simulink model "PTControl"  (Simulink 7.9)
settings: Solver=ode45  StartTime=0.0  StopTime=inf  RelTol=1e-3
PreLoadFcn:
  | FSE_Parameters
undefined symbols (not defined in the file or in its folder): TC_Decr_Gas, TC_Derivative, TC_Incr_Gas, TC_On, TC_Relay_Off, TC_Relay_On, TV_On, TV_Override
libraries: CarMaker4SL x33, simulink x5, simulink_extras x4
(part 2 of 3)

== system PTControl/CarMaker/IPG Vehicle/CarAndTrailer/Trailer/CreateBus Vhcl.Wheel.FL ==
  In1 : Inport
  Bus Creator3 : BusCreator  Inputs=14
  Demux3 : Demux  Outputs=14
  Out1 : Outport
  wires:
  Demux3/1 -> Bus Creator3/1  "Vhcl Wheel FL t x"
  Bus Creator3/1 -> Out1/1
  In1/1 -> Demux3/1
  Demux3/2 -> Bus Creator3/2  "Vhcl Wheel FL t y"
  Demux3/3 -> Bus Creator3/3  "Vhcl Wheel FL t z"
  Demux3/4 -> Bus Creator3/4  "Vhcl Wheel FL r_zxy x"
  Demux3/5 -> Bus Creator3/5  "Vhcl Wheel FL r_zxy y"
  Demux3/6 -> Bus Creator3/6  "Vhcl Wheel FL r_zxy z"
  Demux3/7 -> Bus Creator3/7  "Vhcl Wheel FL Fx"
  Demux3/8 -> Bus Creator3/8  "Vhcl Wheel FL Fy"
  Demux3/9 -> Bus Creator3/9  "Vhcl Wheel FL Fz"
  Demux3/10 -> Bus Creator3/10  "Vhcl Wheel FL vBelt"
  Demux3/11 -> Bus Creator3/11  "Vhcl Wheel FL LongSlip"
  Demux3/12 -> Bus Creator3/12  "Vhcl Wheel FL SideSlip"
  Demux3/13 -> Bus Creator3/13  "Vhcl Wheel FL Trq_T2W"
  Demux3/14 -> Bus Creator3/14  "Vhcl Wheel FL Trq_WhlBearing"

== system PTControl/CarMaker/IPG Vehicle/CarAndTrailer/Trailer/CreateBus Vhcl.Wheel.FR ==
  In1 : Inport
  Bus Creator3 : BusCreator  Inputs=14
  Demux3 : Demux  Outputs=14
  Out1 : Outport
  wires:
  Demux3/1 -> Bus Creator3/1  "Vhcl Wheel FR t x"
  Bus Creator3/1 -> Out1/1
  In1/1 -> Demux3/1
  Demux3/2 -> Bus Creator3/2  "Vhcl Wheel FR t y"
  Demux3/3 -> Bus Creator3/3  "Vhcl Wheel FR t z"
  Demux3/4 -> Bus Creator3/4  "Vhcl Wheel FR r_zxy x"
  Demux3/5 -> Bus Creator3/5  "Vhcl Wheel FR r_zxy y"
  Demux3/6 -> Bus Creator3/6  "Vhcl Wheel FR r_zxy z"
  Demux3/7 -> Bus Creator3/7  "Vhcl Wheel FR Fx"
  Demux3/8 -> Bus Creator3/8  "Vhcl Wheel FR Fy"
  Demux3/9 -> Bus Creator3/9  "Vhcl Wheel FR Fz"
  Demux3/10 -> Bus Creator3/10  "Vhcl Wheel FR vBelt"
  Demux3/11 -> Bus Creator3/11  "Vhcl Wheel FR LongSlip"
  Demux3/12 -> Bus Creator3/12  "Vhcl Wheel FR SideSlip"
  Demux3/13 -> Bus Creator3/13  "Vhcl Wheel FR Trq_T2W"
  Demux3/14 -> Bus Creator3/14  "Vhcl Wheel FR Trq_WhlBearing"

== system PTControl/CarMaker/IPG Vehicle/CarAndTrailer/Trailer/CreateBus Vhcl.Wheel.RL ==
  In1 : Inport
  Bus Creator3 : BusCreator  Inputs=14
  Demux3 : Demux  Outputs=14
  Out1 : Outport
  wires:
  Demux3/1 -> Bus Creator3/1  "Vhcl Wheel RL t x"
  Bus Creator3/1 -> Out1/1
  In1/1 -> Demux3/1
  Demux3/2 -> Bus Creator3/2  "Vhcl Wheel RL t y"
  Demux3/3 -> Bus Creator3/3  "Vhcl Wheel RL t z"
  Demux3/4 -> Bus Creator3/4  "Vhcl Wheel RL r_zxy x"
  Demux3/5 -> Bus Creator3/5  "Vhcl Wheel RL r_zxy y"
  Demux3/6 -> Bus Creator3/6  "Vhcl Wheel RL r_zxy z"
  Demux3/7 -> Bus Creator3/7  "Vhcl Wheel RL Fx"
  Demux3/8 -> Bus Creator3/8  "Vhcl Wheel RL Fy"
  Demux3/9 -> Bus Creator3/9  "Vhcl Wheel RL Fz"
  Demux3/10 -> Bus Creator3/10  "Vhcl Wheel RL vBelt"
  Demux3/11 -> Bus Creator3/11  "Vhcl Wheel RL LongSlip"
  Demux3/12 -> Bus Creator3/12  "Vhcl Wheel RL SideSlip"
  Demux3/13 -> Bus Creator3/13  "Vhcl Wheel RL Trq_T2W"
  Demux3/14 -> Bus Creator3/14  "Vhcl Wheel RL Trq_WhlBearing"

== system PTControl/CarMaker/IPG Vehicle/CarAndTrailer/Trailer/CreateBus Vhcl.Wheel.RR ==
  In1 : Inport
  Bus Creator3 : BusCreator  Inputs=14
  Demux3 : Demux  Outputs=14
  Out1 : Outport
  wires:
  Demux3/1 -> Bus Creator3/1  "Vhcl Wheel RR t x"
  Bus Creator3/1 -> Out1/1
  In1/1 -> Demux3/1
  Demux3/2 -> Bus Creator3/2  "Vhcl Wheel RR t y"
  Demux3/3 -> Bus Creator3/3  "Vhcl Wheel RR t z"
  Demux3/4 -> Bus Creator3/4  "Vhcl Wheel RR r_zxy x"
  Demux3/5 -> Bus Creator3/5  "Vhcl Wheel RR r_zxy y"
  Demux3/6 -> Bus Creator3/6  "Vhcl Wheel RR r_zxy z"
  Demux3/7 -> Bus Creator3/7  "Vhcl Wheel RR Fx"
  Demux3/8 -> Bus Creator3/8  "Vhcl Wheel RR Fy"
  Demux3/9 -> Bus Creator3/9  "Vhcl Wheel RR Fz"
  Demux3/10 -> Bus Creator3/10  "Vhcl Wheel RR vBelt"
  Demux3/11 -> Bus Creator3/11  "Vhcl Wheel RR LongSlip"
  Demux3/12 -> Bus Creator3/12  "Vhcl Wheel RR SideSlip"
  Demux3/13 -> Bus Creator3/13  "Vhcl Wheel RR Trq_T2W"
  Demux3/14 -> Bus Creator3/14  "Vhcl Wheel RR Trq_WhlBearing"

== system PTControl/CarMaker/IPG Vehicle/PowerTrain/PTControl Example/CreateBus PTC ClutchOut ==
  In : Inport
  BusCreator : BusCreator  Inputs=3
  Demux : Demux  Outputs=3
  Out : Outport
  wires:
  In/1 -> Demux/1
  BusCreator/1 -> Out/1
  Demux/1 -> BusCreator/1  "PTC ClutchOut Pos"
  Demux/2 -> BusCreator/2  "PTC ClutchOut rotv_out_trg"
  Demux/3 -> BusCreator/3  "PTC ClutchOut Trq_out_trg"

== system PTControl/CarMaker/IPG Vehicle/PowerTrain/PTControl Example/CreateBus PTC EngineOut ==
  In : Inport
  BusCreator : BusCreator  Inputs=5
  Demux : Demux  Outputs=5
  Out : Outport
  wires:
  In/1 -> Demux/1
  BusCreator/1 -> Out/1
  Demux/1 -> BusCreator/1  "PTC EngineOut set_ISC"
  Demux/2 -> BusCreator/2  "PTC EngineOut FuelCutOff"
  Demux/3 -> BusCreator/3  "PTC EngineOut Load"
  Demux/4 -> BusCreator/4  "PTC EngineOut Trq_trg"
  Demux/5 -> BusCreator/5  "PTC EngineOut rotv_trg"

== system PTControl/CarMaker/IPG Vehicle/PowerTrain/PTControl Example/CreateBus PTC GearBoxM_Out0 ==
  In : Inport
  BusCreator : BusCreator  Inputs=7
  Demux : Demux  Outputs=7
  Out : Outport
  wires:
  In/1 -> Demux/1
  BusCreator/1 -> Out/1
  Demux/1 -> BusCreator/1  "PTC GearBoxM_Out0 GearNoTrg"
  Demux/2 -> BusCreator/2  "PTC GearBoxM_Out0 set_ParkBrake"
  Demux/3 -> BusCreator/3  "PTC GearBoxM_Out0 rotv_in_trg"
  Demux/4 -> BusCreator/4  "PTC GearBoxM_Out0 Trq_out_trg"
  Demux/5 -> BusCreator/5  "PTC GearBoxM_Out0 Clutch Pos"
  Demux/6 -> BusCreator/6  "PTC GearBoxM_Out0 Clutch rotv_out_trg"
  Demux/7 -> BusCreator/7  "PTC GearBoxM_Out0 Clutch Trq_out_trg"

== system PTControl/CarMaker/IPG Vehicle/PowerTrain/PTControl Example/CreateBus PTC GearBoxM_Out1 ==
  In : Inport
  BusCreator : BusCreator  Inputs=7
  Demux : Demux  Outputs=7
  Out : Outport
  wires:
  In/1 -> Demux/1
  BusCreator/1 -> Out/1
  Demux/1 -> BusCreator/1  "PTC GearBoxM_Out1 GearNoTrg"
  Demux/2 -> BusCreator/2  "PTC GearBoxM_Out1 set_ParkBrake"
  Demux/3 -> BusCreator/3  "PTC GearBoxM_Out1 rotv_in_trg"
  Demux/4 -> BusCreator/4  "PTC GearBoxM_Out1 Trq_out_trg"
  Demux/5 -> BusCreator/5  "PTC GearBoxM_Out1 Clutch Pos"
  Demux/6 -> BusCreator/6  "PTC GearBoxM_Out1 Clutch rotv_out_trg"
  Demux/7 -> BusCreator/7  "PTC GearBoxM_Out1 Clutch Trq_out_trg"

== system PTControl/CarMaker/IPG Vehicle/PowerTrain/PTControl Example/CreateBus PTC GearBoxM_Out2 ==
  In : Inport
  BusCreator : BusCreator  Inputs=7
  Demux : Demux  Outputs=7
  Out : Outport
  wires:
  In/1 -> Demux/1
  BusCreator/1 -> Out/1
  Demux/1 -> BusCreator/1  "PTC GearBoxM_Out2 GearNoTrg"
  Demux/2 -> BusCreator/2  "PTC GearBoxM_Out2 set_ParkBrake"
  Demux/3 -> BusCreator/3  "PTC GearBoxM_Out2 rotv_in_trg"
  Demux/4 -> BusCreator/4  "PTC GearBoxM_Out2 Trq_out_trg"
  Demux/5 -> BusCreator/5  "PTC GearBoxM_Out2 Clutch Pos"
  Demux/6 -> BusCreator/6  "PTC GearBoxM_Out2 Clutch rotv_out_trg"
  Demux/7 -> BusCreator/7  "PTC GearBoxM_Out2 Clutch Trq_out_trg"

== system PTControl/CarMaker/IPG Vehicle/PowerTrain/PTControl Example/CreateBus PTC GearBoxM_Out3 ==
  In : Inport
  BusCreator : BusCreator  Inputs=7
  Demux : Demux  Outputs=7
  Out : Outport
  wires:
  In/1 -> Demux/1
  BusCreator/1 -> Out/1
  Demux/1 -> BusCreator/1  "PTC GearBoxM_Out3 GearNoTrg"
  Demux/2 -> BusCreator/2  "PTC GearBoxM_Out3 set_ParkBrake"
  Demux/3 -> BusCreator/3  "PTC GearBoxM_Out3 rotv_in_trg"
  Demux/4 -> BusCreator/4  "PTC GearBoxM_Out3 Trq_out_trg"
  Demux/5 -> BusCreator/5  "PTC GearBoxM_Out3 Clutch Pos"
  Demux/6 -> BusCreator/6  "PTC GearBoxM_Out3 Clutch rotv_out_trg"
  Demux/7 -> BusCreator/7  "PTC GearBoxM_Out3 Clutch Trq_out_trg"

== system PTControl/CarMaker/IPG Vehicle/PowerTrain/PTControl Example/CreateBus PTC GearBoxOut ==
  In : Inport
  BusCreator : BusCreator  Inputs=7
  Demux : Demux  Outputs=7
  Out : Outport
  wires:
  In/1 -> Demux/1
  BusCreator/1 -> Out/1
  Demux/1 -> BusCreator/1  "PTC GearBoxOut GearNoTrg"
  Demux/2 -> BusCreator/2  "PTC GearBoxOut set_ParkBrake"
  Demux/3 -> BusCreator/3  "PTC GearBoxOut rotv_in_trg"
  Demux/4 -> BusCreator/4  "PTC GearBoxOut Trq_out_trg"
  Demux/5 -> BusCreator/5  "PTC GearBoxOut Clutch Pos"
  Demux/6 -> BusCreator/6  "PTC GearBoxOut Clutch rotv_out_trg"
  Demux/7 -> BusCreator/7  "PTC GearBoxOut Clutch Trq_out_trg"

== system PTControl/CarMaker/IPG Vehicle/PowerTrain/PTControl Example/CreateBus PTC ISGOut ==
  In : Inport
  BusCreator : BusCreator  Inputs=3
  Demux : Demux  Outputs=3
  Out : Outport
  wires:
  In/1 -> Demux/1
  BusCreator/1 -> Out/1
  Demux/1 -> BusCreator/1  "PTC ISGOut Load"
  Demux/2 -> BusCreator/2  "PTC ISGOut Trq_trg"
  Demux/3 -> BusCreator/3  "PTC ISGOut rotv_trg"

== system PTControl/CarMaker/IPG Vehicle/PowerTrain/PTControl Example/CreateBus PTC MiscOut ==
  In : Inport
  BusCreator : BusCreator
  Demux : Demux
  Out : Outport
  wires:
  In/1 -> Demux/1
  BusCreator/1 -> Out/1
  Demux/1 -> BusCreator/1  "PTC_Out OperationState"
  Demux/2 -> BusCreator/2  "PTC_Out OperationError"
  Demux/3 -> BusCreator/3  "PTC_Out StrategyMode"
  Demux/4 -> BusCreator/4  "PTC_Out Ignition"

== system PTControl/CarMaker/IPG Vehicle/PowerTrain/PTControl Example/CreateBus PTC MotorOut0 ==
  In : Inport
  BusCreator : BusCreator  Inputs=3
  Demux : Demux  Outputs=3
  Out : Outport
  wires:
  In/1 -> Demux/1
  BusCreator/1 -> Out/1
  Demux/1 -> BusCreator/1  "PTC MotorOut0 Load"
  Demux/2 -> BusCreator/2  "PTC MotorOut0 Trq_trg"
  Demux/3 -> BusCreator/3  "PTC MotorOut0 rotv_trg"

== system PTControl/CarMaker/IPG Vehicle/PowerTrain/PTControl Example/CreateBus PTC MotorOut1 ==
  In : Inport
  BusCreator : BusCreator  Inputs=3
  Demux : Demux  Outputs=3
  Out : Outport
  wires:
  In/1 -> Demux/1
  BusCreator/1 -> Out/1
  Demux/1 -> BusCreator/1  "PTC MotorOut1 Load"
  Demux/2 -> BusCreator/2  "PTC MotorOut1 Trq_trg"
  Demux/3 -> BusCreator/3  "PTC MotorOut1 rotv_trg"

== system PTControl/CarMaker/IPG Vehicle/PowerTrain/PTControl Example/CreateBus PTC MotorOut2 ==
  In : Inport
  BusCreator : BusCreator  Inputs=3
  Demux : Demux  Outputs=3
  Out : Outport
  wires:
  In/1 -> Demux/1
  BusCreator/1 -> Out/1
  Demux/1 -> BusCreator/1  "PTC MotorOut2 Load"
  Demux/2 -> BusCreator/2  "PTC MotorOut2 Trq_trg"
  Demux/3 -> BusCreator/3  "PTC MotorOut2 rotv_trg"

== system PTControl/CarMaker/IPG Vehicle/PowerTrain/PTControl Example/CreateBus PTC MotorOut3 ==
  In : Inport
  BusCreator : BusCreator  Inputs=3
  Demux : Demux  Outputs=3
  Out : Outport
  wires:
  In/1 -> Demux/1
  BusCreator/1 -> Out/1
  Demux/1 -> BusCreator/1  "PTC MotorOut3 Load"
  Demux/2 -> BusCreator/2  "PTC MotorOut3 Trq_trg"
  Demux/3 -> BusCreator/3  "PTC MotorOut3 rotv_trg"

== system PTControl/CarMaker/IPG Vehicle/PowerTrain/PTControl Example/CreateBus PTC PwrSupplyOut ==
  In : Inport
  BusCreator : BusCreator  Inputs=1
  Demux : Demux  Outputs=1
  Out : Outport
  wires:
  In/1 -> Demux/1
  BusCreator/1 -> Out/1
  Demux/1 -> BusCreator/1  "PTC PwrSupplyOut Pwr_HV1toLV_trg"

== system PTControl/CarMaker/IPG Vehicle/PowerTrain/PTControl Example/CreateBus PTC WheelOut ==
  In : Inport
  BusCreator : BusCreator  Inputs=8
  Demux : Demux  Outputs=8
  Out : Outport
  wires:
  In/1 -> Demux/1
  BusCreator/1 -> Out/1
  Demux/1 -> BusCreator/1  "PTC WheelOut_FL Trq_BrakeReg"
  Demux/2 -> BusCreator/2  "PTC WheelOut_FL Trq_BrakeReg_max"
  Demux/3 -> BusCreator/3  "PTC WheelOut_FR Trq_BrakeReg"
  Demux/4 -> BusCreator/4  "PTC WheelOut_FR Trq_BrakeReg_max"
  Demux/5 -> BusCreator/5  "PTC WheelOut_RL Trq_BrakeReg"
  Demux/6 -> BusCreator/6  "PTC WheelOut_RL Trq_BrakeReg_max"
  Demux/7 -> BusCreator/7  "PTC WheelOut_RR Trq_BrakeReg"
  Demux/8 -> BusCreator/8  "PTC WheelOut_RR Trq_BrakeReg_max"

== system PTControl/CarMaker/IPG Vehicle/PowerTrain/PTControl Example/PTControl Example ==
  note: Minimalistic PTControl example model to be used with
      | FS_RaceCar_5.1_electric_TorqueVectoring
  VhclCtrl.PT : Inport
  Bus Selector : BusSelector  OutputSignals=VhclCtrl Gas
  PTC : Subsystem
  Torque Control 0 : Subsystem
  Torque Control 1 : Subsystem
  Torque Control 2 : Subsystem
  Torque Control 3 : Subsystem
  PTC MiscOut : Outport
  MotorOut0 : Outport  Port=2
  MotorOut1 : Outport  Port=3
  MotorOut2 : Outport  Port=4
  MotorOut3 : Outport  Port=5
  wires:
  PTC/1(PTC MiscOut) -> PTC MiscOut/1
  VhclCtrl.PT/1 -> Bus Selector/1
  Torque Control 0/1(MotorOut0) -> MotorOut0/1
  Torque Control 1/1(MotorOut1) -> MotorOut1/1
  Torque Control 2/1(MotorOut2) -> MotorOut2/1
  Torque Control 3/1(MotorOut3) -> MotorOut3/1
  Bus Selector/1 -> Torque Control 1/1(Gas), Torque Control 0/1(Gas), Torque Control 2/1(Gas), Torque Control 3/1(Gas)  "<VhclCtrl Gas>"

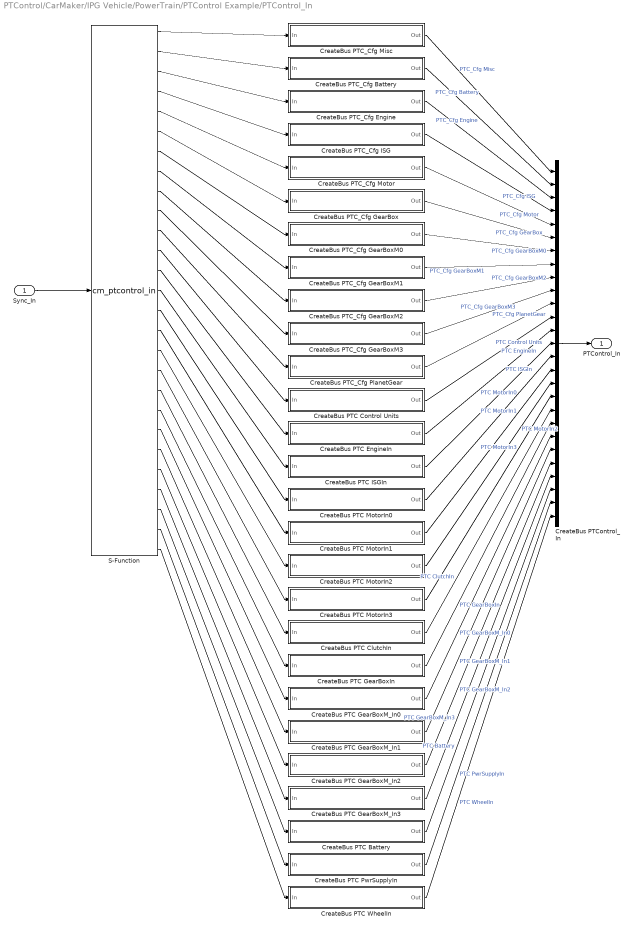
== system PTControl/CarMaker/IPG Vehicle/PowerTrain/PTControl Example/PTControl_In ==
  Sync_In : Inport
  CreateBus PTC Battery : Subsystem
  CreateBus PTC ClutchIn : Subsystem
  CreateBus PTC Control Units : Subsystem
  CreateBus PTC EngineIn : Subsystem
  CreateBus PTC GearBoxIn : Subsystem
  CreateBus PTC GearBoxM_In0 : Subsystem
  CreateBus PTC GearBoxM_In1 : Subsystem
  CreateBus PTC GearBoxM_In2 : Subsystem
  CreateBus PTC GearBoxM_In3 : Subsystem
  CreateBus PTC ISGIn : Subsystem
  CreateBus PTC MotorIn0 : Subsystem
  CreateBus PTC MotorIn1 : Subsystem
  CreateBus PTC MotorIn2 : Subsystem
  CreateBus PTC MotorIn3 : Subsystem
  CreateBus PTC PwrSupplyIn : Subsystem
  CreateBus PTC WheelIn : Subsystem
  CreateBus PTC_Cfg Battery : Subsystem
  CreateBus PTC_Cfg Engine : Subsystem
  CreateBus PTC_Cfg GearBox : Subsystem
  CreateBus PTC_Cfg GearBoxM0 : Subsystem
  CreateBus PTC_Cfg GearBoxM1 : Subsystem
  CreateBus PTC_Cfg GearBoxM2 : Subsystem
  CreateBus PTC_Cfg GearBoxM3 : Subsystem
  CreateBus PTC_Cfg ISG : Subsystem
  CreateBus PTC_Cfg Misc : Subsystem
  CreateBus PTC_Cfg Motor : Subsystem
  CreateBus PTC_Cfg PlanetGear : Subsystem
  CreateBus PTControl_In : BusCreator  Inputs=27
  S-Function : S-Function  FunctionName=cm_ptcontrol_in  EnableBusSupport=off
  PTControl_In : Outport
  wires:
  Sync_In/1 -> S-Function/1
  CreateBus PTControl_In/1 -> PTControl_In/1
  S-Function/1 -> CreateBus PTC_Cfg Misc/1(In)
  CreateBus PTC_Cfg Misc/1(Out) -> CreateBus PTControl_In/1  "PTC_Cfg Misc"
  S-Function/2 -> CreateBus PTC_Cfg Battery/1(In)
  CreateBus PTC_Cfg Battery/1(Out) -> CreateBus PTControl_In/2  "PTC_Cfg Battery"
  S-Function/3 -> CreateBus PTC_Cfg Engine/1(In)
  CreateBus PTC_Cfg Engine/1(Out) -> CreateBus PTControl_In/3  "PTC_Cfg Engine"
  S-Function/4 -> CreateBus PTC_Cfg ISG/1(In)
  CreateBus PTC_Cfg ISG/1(Out) -> CreateBus PTControl_In/4  "PTC_Cfg ISG"
  S-Function/5 -> CreateBus PTC_Cfg Motor/1(In)
  CreateBus PTC_Cfg Motor/1(Out) -> CreateBus PTControl_In/5  "PTC_Cfg Motor"
  S-Function/6 -> CreateBus PTC_Cfg GearBox/1(In)
  CreateBus PTC_Cfg GearBox/1(Out) -> CreateBus PTControl_In/6  "PTC_Cfg GearBox"
  S-Function/7 -> CreateBus PTC_Cfg GearBoxM0/1(In)
  CreateBus PTC_Cfg GearBoxM0/1(Out) -> CreateBus PTControl_In/7  "PTC_Cfg GearBoxM0"
  S-Function/8 -> CreateBus PTC_Cfg GearBoxM1/1(In)
  CreateBus PTC_Cfg GearBoxM1/1(Out) -> CreateBus PTControl_In/8  "PTC_Cfg GearBoxM1"
  S-Function/9 -> CreateBus PTC_Cfg GearBoxM2/1(In)
  CreateBus PTC_Cfg GearBoxM2/1(Out) -> CreateBus PTControl_In/9  "PTC_Cfg GearBoxM2"
  S-Function/10 -> CreateBus PTC_Cfg GearBoxM3/1(In)
  CreateBus PTC_Cfg GearBoxM3/1(Out) -> CreateBus PTControl_In/10  "PTC_Cfg GearBoxM3"
  S-Function/11 -> CreateBus PTC_Cfg PlanetGear/1(In)
  CreateBus PTC_Cfg PlanetGear/1(Out) -> CreateBus PTControl_In/11  "PTC_Cfg PlanetGear"
  S-Function/12 -> CreateBus PTC Control Units/1(In)
  CreateBus PTC Control Units/1(Out) -> CreateBus PTControl_In/12  "PTC Control Units"
  S-Function/13 -> CreateBus PTC EngineIn/1(In)
  CreateBus PTC EngineIn/1(Out) -> CreateBus PTControl_In/13  "PTC EngineIn"
  S-Function/14 -> CreateBus PTC ISGIn/1(In)
  CreateBus PTC ISGIn/1(Out) -> CreateBus PTControl_In/14  "PTC ISGIn"
  S-Function/15 -> CreateBus PTC MotorIn0/1(In)
  CreateBus PTC MotorIn0/1(Out) -> CreateBus PTControl_In/15  "PTC MotorIn0"
  S-Function/16 -> CreateBus PTC MotorIn1/1(In)
  CreateBus PTC MotorIn1/1(Out) -> CreateBus PTControl_In/16  "PTC MotorIn1"
  S-Function/17 -> CreateBus PTC MotorIn2/1(In)
  CreateBus PTC MotorIn2/1(Out) -> CreateBus PTControl_In/17  "PTC MotorIn2"
  S-Function/18 -> CreateBus PTC MotorIn3/1(In)
  CreateBus PTC MotorIn3/1(Out) -> CreateBus PTControl_In/18  "PTC MotorIn3"
  S-Function/19 -> CreateBus PTC ClutchIn/1(In)
  CreateBus PTC ClutchIn/1(Out) -> CreateBus PTControl_In/19  "PTC ClutchIn"
  S-Function/20 -> CreateBus PTC GearBoxIn/1(In)
  CreateBus PTC GearBoxIn/1(Out) -> CreateBus PTControl_In/20  "PTC GearBoxIn"
  S-Function/21 -> CreateBus PTC GearBoxM_In0/1(In)
  CreateBus PTC GearBoxM_In0/1(Out) -> CreateBus PTControl_In/21  "PTC GearBoxM_In0"
  S-Function/22 -> CreateBus PTC GearBoxM_In1/1(In)
  CreateBus PTC GearBoxM_In1/1(Out) -> CreateBus PTControl_In/22  "PTC GearBoxM_In1"
  S-Function/23 -> CreateBus PTC GearBoxM_In2/1(In)
  CreateBus PTC GearBoxM_In2/1(Out) -> CreateBus PTControl_In/23  "PTC GearBoxM_In2"
  S-Function/24 -> CreateBus PTC GearBoxM_In3/1(In)
  CreateBus PTC GearBoxM_In3/1(Out) -> CreateBus PTControl_In/24  "PTC GearBoxM_In3"
  S-Function/25 -> CreateBus PTC Battery/1(In)
  CreateBus PTC Battery/1(Out) -> CreateBus PTControl_In/25  "PTC Battery"
  S-Function/26 -> CreateBus PTC PwrSupplyIn/1(In)
  CreateBus PTC PwrSupplyIn/1(Out) -> CreateBus PTControl_In/26  "PTC PwrSupplyIn"
  S-Function/27 -> CreateBus PTC WheelIn/1(In)
  CreateBus PTC WheelIn/1(Out) -> CreateBus PTControl_In/27  "PTC WheelIn"

== system PTControl/CarMaker/IPG Vehicle/PowerTrain/PTControl Example/PTControl_Out ==
  PTC MiscOut : Inport
  PTC EngineOut : Inport  Port=2
  PTC ISGOut : Inport  Port=3
  PTC MotorOut0 : Inport  Port=4
  PTC MotorOut1 : Inport  Port=5
  PTC MotorOut2 : Inport  Port=6
  PTC MotorOut3 : Inport  Port=7
  PTC ClutchOut : Inport  Port=8
  PTC GearBoxOut : Inport  Port=9
  PTC GearBoxM_Out0 : Inport  Port=10
  PTC GearBoxM_Out1 : Inport  Port=11
  PTC GearBoxM_Out2 : Inport  Port=12
  PTC GearBoxM_Out3 : Inport  Port=13
  PTC PwrSupplyOut : Inport  Port=14
  PTC WheelOut : Inport  Port=15
  PTControl_Out : S-Function  FunctionName=cm_ptcontrol_out  EnableBusSupport=off
  wires:
  PTC MiscOut/1 -> PTControl_Out/1
  PTC EngineOut/1 -> PTControl_Out/2
  PTC ISGOut/1 -> PTControl_Out/3
  PTC MotorOut0/1 -> PTControl_Out/4
  PTC MotorOut1/1 -> PTControl_Out/5
  PTC MotorOut2/1 -> PTControl_Out/6
  PTC MotorOut3/1 -> PTControl_Out/7
  PTC ClutchOut/1 -> PTControl_Out/8
  PTC GearBoxOut/1 -> PTControl_Out/9
  PTC GearBoxM_Out0/1 -> PTControl_Out/10
  PTC GearBoxM_Out1/1 -> PTControl_Out/11
  PTC GearBoxM_Out2/1 -> PTControl_Out/12
  PTC GearBoxM_Out3/1 -> PTControl_Out/13
  PTC PwrSupplyOut/1 -> PTControl_Out/14
  PTC WheelOut/1 -> PTControl_Out/15

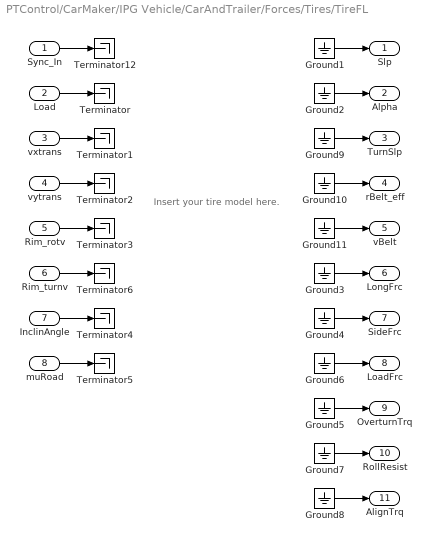
== system PTControl/CarMaker/IPG Vehicle/CarAndTrailer/Forces/Tires/TireFL ==
  note: Insert your tire model here.
  Sync_In : Inport
  Load : Inport  Port=2
  vxtrans : Inport  Port=3
  vytrans : Inport  Port=4
  Rim_rotv : Inport  Port=5
  Rim_turnv : Inport  Port=6
  InclinAngle : Inport  Port=7
  muRoad : Inport  Port=8
  Ground{1..11} (11 alike) : Ground
  Terminator{,1..6,12} (8 alike) : Terminator
  Slp : Outport
  Alpha : Outport  Port=2
  TurnSlp : Outport  Port=3
  rBelt_eff : Outport  Port=4
  vBelt : Outport  Port=5
  LongFrc : Outport  Port=6
  SideFrc : Outport  Port=7
  LoadFrc : Outport  Port=8
  OverturnTrq : Outport  Port=9
  RollResist : Outport  Port=10
  AlignTrq : Outport  Port=11
  wires:
  Ground11/1 -> vBelt/1
  Ground10/1 -> rBelt_eff/1
  Ground9/1 -> TurnSlp/1
  Rim_turnv/1 -> Terminator6/1
  Sync_In/1 -> Terminator12/1
  Ground2/1 -> Alpha/1
  Ground3/1 -> LongFrc/1
  Ground4/1 -> SideFrc/1
  Ground5/1 -> OverturnTrq/1
  vxtrans/1 -> Terminator1/1
  vytrans/1 -> Terminator2/1
  Rim_rotv/1 -> Terminator3/1
  InclinAngle/1 -> Terminator4/1
  muRoad/1 -> Terminator5/1
  Load/1 -> Terminator/1
  Ground1/1 -> Slp/1
  Ground6/1 -> LoadFrc/1
  Ground7/1 -> RollResist/1
  Ground8/1 -> AlignTrq/1

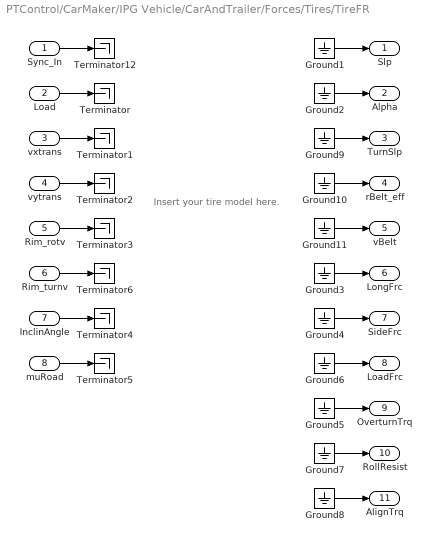
== system PTControl/CarMaker/IPG Vehicle/CarAndTrailer/Forces/Tires/TireFR ==
  note: Insert your tire model here.
  Sync_In : Inport
  Load : Inport  Port=2
  vxtrans : Inport  Port=3
  vytrans : Inport  Port=4
  Rim_rotv : Inport  Port=5
  Rim_turnv : Inport  Port=6
  InclinAngle : Inport  Port=7
  muRoad : Inport  Port=8
  Ground{1..11} (11 alike) : Ground
  Terminator{,1..6,12} (8 alike) : Terminator
  Slp : Outport
  Alpha : Outport  Port=2
  TurnSlp : Outport  Port=3
  rBelt_eff : Outport  Port=4
  vBelt : Outport  Port=5
  LongFrc : Outport  Port=6
  SideFrc : Outport  Port=7
  LoadFrc : Outport  Port=8
  OverturnTrq : Outport  Port=9
  RollResist : Outport  Port=10
  AlignTrq : Outport  Port=11
  wires:
  Ground11/1 -> vBelt/1
  Ground10/1 -> rBelt_eff/1
  Ground9/1 -> TurnSlp/1
  Rim_turnv/1 -> Terminator6/1
  Sync_In/1 -> Terminator12/1
  Ground2/1 -> Alpha/1
  Ground3/1 -> LongFrc/1
  Ground4/1 -> SideFrc/1
  Ground5/1 -> OverturnTrq/1
  vxtrans/1 -> Terminator1/1
  vytrans/1 -> Terminator2/1
  Rim_rotv/1 -> Terminator3/1
  InclinAngle/1 -> Terminator4/1
  muRoad/1 -> Terminator5/1
  Load/1 -> Terminator/1
  Ground1/1 -> Slp/1
  Ground6/1 -> LoadFrc/1
  Ground7/1 -> RollResist/1
  Ground8/1 -> AlignTrq/1

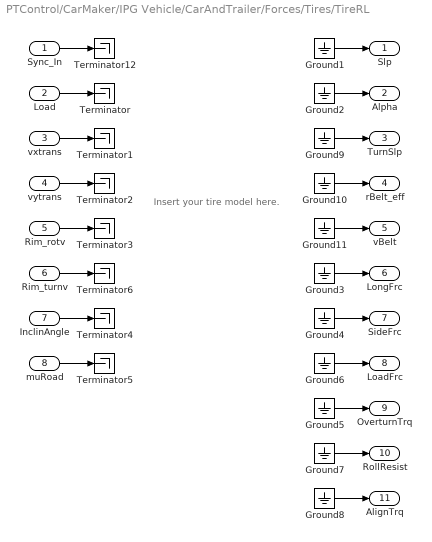
== system PTControl/CarMaker/IPG Vehicle/CarAndTrailer/Forces/Tires/TireRL ==
  note: Insert your tire model here.
  Sync_In : Inport
  Load : Inport  Port=2
  vxtrans : Inport  Port=3
  vytrans : Inport  Port=4
  Rim_rotv : Inport  Port=5
  Rim_turnv : Inport  Port=6
  InclinAngle : Inport  Port=7
  muRoad : Inport  Port=8
  Ground{1..11} (11 alike) : Ground
  Terminator{,1..6,12} (8 alike) : Terminator
  Slp : Outport
  Alpha : Outport  Port=2
  TurnSlp : Outport  Port=3
  rBelt_eff : Outport  Port=4
  vBelt : Outport  Port=5
  LongFrc : Outport  Port=6
  SideFrc : Outport  Port=7
  LoadFrc : Outport  Port=8
  OverturnTrq : Outport  Port=9
  RollResist : Outport  Port=10
  AlignTrq : Outport  Port=11
  wires:
  Ground11/1 -> vBelt/1
  Ground10/1 -> rBelt_eff/1
  Ground9/1 -> TurnSlp/1
  Rim_turnv/1 -> Terminator6/1
  Sync_In/1 -> Terminator12/1
  Ground2/1 -> Alpha/1
  Ground3/1 -> LongFrc/1
  Ground4/1 -> SideFrc/1
  Ground5/1 -> OverturnTrq/1
  vxtrans/1 -> Terminator1/1
  vytrans/1 -> Terminator2/1
  Rim_rotv/1 -> Terminator3/1
  InclinAngle/1 -> Terminator4/1
  muRoad/1 -> Terminator5/1
  Load/1 -> Terminator/1
  Ground1/1 -> Slp/1
  Ground6/1 -> LoadFrc/1
  Ground7/1 -> RollResist/1
  Ground8/1 -> AlignTrq/1

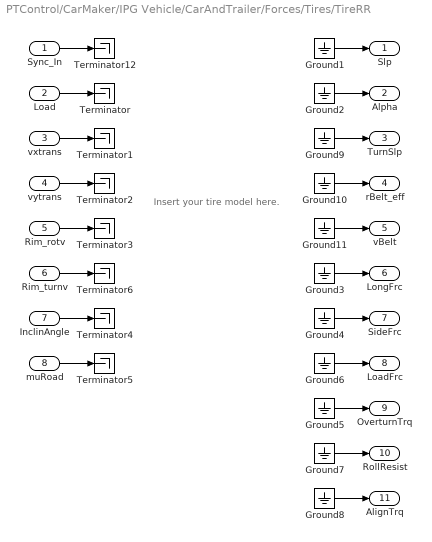
== system PTControl/CarMaker/IPG Vehicle/CarAndTrailer/Forces/Tires/TireRR ==
  note: Insert your tire model here.
  Sync_In : Inport
  Load : Inport  Port=2
  vxtrans : Inport  Port=3
  vytrans : Inport  Port=4
  Rim_rotv : Inport  Port=5
  Rim_turnv : Inport  Port=6
  InclinAngle : Inport  Port=7
  muRoad : Inport  Port=8
  Ground{1..11} (11 alike) : Ground
  Terminator{,1..6,12} (8 alike) : Terminator
  Slp : Outport
  Alpha : Outport  Port=2
  TurnSlp : Outport  Port=3
  rBelt_eff : Outport  Port=4
  vBelt : Outport  Port=5
  LongFrc : Outport  Port=6
  SideFrc : Outport  Port=7
  LoadFrc : Outport  Port=8
  OverturnTrq : Outport  Port=9
  RollResist : Outport  Port=10
  AlignTrq : Outport  Port=11
  wires:
  Ground11/1 -> vBelt/1
  Ground10/1 -> rBelt_eff/1
  Ground9/1 -> TurnSlp/1
  Rim_turnv/1 -> Terminator6/1
  Sync_In/1 -> Terminator12/1
  Ground2/1 -> Alpha/1
  Ground3/1 -> LongFrc/1
  Ground4/1 -> SideFrc/1
  Ground5/1 -> OverturnTrq/1
  vxtrans/1 -> Terminator1/1
  vytrans/1 -> Terminator2/1
  Rim_rotv/1 -> Terminator3/1
  InclinAngle/1 -> Terminator4/1
  muRoad/1 -> Terminator5/1
  Load/1 -> Terminator/1
  Ground1/1 -> Slp/1
  Ground6/1 -> LoadFrc/1
  Ground7/1 -> RollResist/1
  Ground8/1 -> AlignTrq/1

== system PTControl/CarMaker/IPG Vehicle/PowerTrain/PTControl Example/PTControl Example/PTC ==
  Constant : Constant
  Ground : Ground
  Mode_ElectricDrive : Constant  Value=4
  Mux : Mux
  OperState_Driving : Constant  Value=4
  PTC MiscOut : Outport
  wires:
  Mode_ElectricDrive/1 -> Mux/3
  OperState_Driving/1 -> Mux/1  "OperationState"
  Mux/1 -> PTC MiscOut/1
  Ground/1 -> Mux/2  "OperationError"
  Constant/1 -> Mux/4  "Ignition"

== system PTControl/CarMaker/IPG Vehicle/PowerTrain/PTControl Example/PTControl Example/Torque Control 0 ==
  note: Trq_trg
  note: Load_Motor0_FL
  Gas : Inport
  Add : Sum
  Constant2 : Constant  Value=TC_On
  Constant4 : Constant  Value=TV_On
  Electronic Gas Pedal FL : Subsystem
  Mux : Mux  Inputs=3
  NOTSET1 : Constant  Value=-99999
  NOTSET3 : Constant  Value=-99999
  Product1 : Product  RndMeth=Zero
  Scope : Scope
  Torque Vectoring FL : Subsystem
  MotorOut0 : Outport
  wires:
  Mux/1 -> MotorOut0/1
  Constant2/1 -> Electronic Gas Pedal FL/1(TV_On)
  Electronic Gas Pedal FL/1(Motor_Gas_FL) -> Add/1
  Torque Vectoring FL/1(TV FL) -> Product1/1
  Constant4/1 -> Product1/2
  Product1/1 -> Add/2
  Add/1 -> Mux/1, Scope/1
  NOTSET3/1 -> Mux/2
  NOTSET1/1 -> Mux/3  "rotv_trg"
  Gas/1 -> Electronic Gas Pedal FL/2(VC.Gas)

== system PTControl/CarMaker/IPG Vehicle/PowerTrain/PTControl Example/PTControl Example/Torque Control 1 ==
  note: Load_Motor1_FR
  note: Trq_trg
  Gas : Inport
  Add : Sum
  Constant2 : Constant  Value=TC_On
  Constant4 : Constant  Value=TV_On
  Electronic Gas Pedal FR : Subsystem
  Mux : Mux  Inputs=3
  NOTSET1 : Constant  Value=-99999
  NOTSET3 : Constant  Value=-99999
  Product1 : Product  RndMeth=Zero
  Torque Vectoring FR : Subsystem
  MotorOut1 : Outport
  wires:
  NOTSET1/1 -> Mux/3  "rotv_trg"
  NOTSET3/1 -> Mux/2
  Add/1 -> Mux/1
  Product1/1 -> Add/2
  Constant4/1 -> Product1/2
  Torque Vectoring FR/1(TV FR) -> Product1/1
  Electronic Gas Pedal FR/1(Motor_Gas_FR) -> Add/1
  Constant2/1 -> Electronic Gas Pedal FR/1(TV_On)
  Mux/1 -> MotorOut1/1
  Gas/1 -> Electronic Gas Pedal FR/2(VC.Gas)

== system PTControl/CarMaker/IPG Vehicle/PowerTrain/PTControl Example/PTControl Example/Torque Control 2 ==
  note: Load_Motor2_RL
  note: Trq_trg
  Gas : Inport
  Add : Sum
  Constant2 : Constant  Value=TC_On
  Constant4 : Constant  Value=TV_On
  Electronic Gas Pedal RL : Subsystem
  Mux : Mux  Inputs=3
  NOTSET1 : Constant  Value=-99999
  NOTSET3 : Constant  Value=-99999
  Product1 : Product  RndMeth=Zero
  Torque Vectoring RL : Subsystem
  MotorOut2 : Outport
  wires:
  NOTSET1/1 -> Mux/3  "rotv_trg"
  NOTSET3/1 -> Mux/2
  Add/1 -> Mux/1
  Product1/1 -> Add/2
  Constant4/1 -> Product1/2
  Torque Vectoring RL/1(TV RL) -> Product1/1
  Electronic Gas Pedal RL/1(Motor_Gas_RL) -> Add/1
  Constant2/1 -> Electronic Gas Pedal RL/1(TV_On)
  Mux/1 -> MotorOut2/1
  Gas/1 -> Electronic Gas Pedal RL/2(VC.Gas)

== system PTControl/CarMaker/IPG Vehicle/PowerTrain/PTControl Example/PTControl Example/Torque Control 3 ==
  note: Trq_trg
  note: Load_Motor3_RR
  Gas : Inport
  Add : Sum
  Constant2 : Constant  Value=TC_On
  Constant4 : Constant  Value=TV_On
  Electronic Gas Pedal RR : Subsystem
  Mux : Mux  Inputs=3
  NOTSET1 : Constant  Value=-99999
  NOTSET3 : Constant  Value=-99999
  Product1 : Product  RndMeth=Zero
  Torque Vectoring RR : Subsystem
  MotorOut3 : Outport
  wires:
  Mux/1 -> MotorOut3/1
  Constant2/1 -> Electronic Gas Pedal RR/1(TV_On)
  Electronic Gas Pedal RR/1(Motor_Gas_RR) -> Add/1
  Torque Vectoring RR/1(TV RR) -> Product1/1
  Constant4/1 -> Product1/2
  Product1/1 -> Add/2
  Add/1 -> Mux/1
  NOTSET3/1 -> Mux/2
  NOTSET1/1 -> Mux/3  "rotv_trg"
  Gas/1 -> Electronic Gas Pedal RR/2(VC.Gas)

== system PTControl/CarMaker/IPG Vehicle/PowerTrain/PTControl Example/PTControl_In/CreateBus PTC Battery ==
  In : Inport
  BusCreator : BusCreator  Inputs=14
  Demux : Demux  Outputs=14
  Out : Outport
  wires:
  In/1 -> Demux/1
  BusCreator/1 -> Out/1
  Demux/1 -> BusCreator/1  "PTC BattLVIn SOC"
  Demux/2 -> BusCreator/2  "PTC BattLVIn SOH"
  Demux/3 -> BusCreator/3  "PTC BattLVIn Current"
  Demux/4 -> BusCreator/4  "PTC BattLVIn AOC"
  Demux/5 -> BusCreator/5  "PTC BattLVIn Temp"
  Demux/6 -> BusCreator/6  "PTC BattLVIn Energy"
  Demux/7 -> BusCreator/7  "PTC BattLVIn Pwr_max"
  Demux/8 -> BusCreator/8  "PTC BattHVIn SOC"
  Demux/9 -> BusCreator/9  "PTC BattHVIn SOH"
  Demux/10 -> BusCreator/10  "PTC BattHVIn Current"
  Demux/11 -> BusCreator/11  "PTC BattHVIn AOC"
  Demux/12 -> BusCreator/12  "PTC BattHVIn Temp"
  Demux/13 -> BusCreator/13  "PTC BattHVIn Energy"
  Demux/14 -> BusCreator/14  "PTC BattHVIn Pwr_max"

== system PTControl/CarMaker/IPG Vehicle/PowerTrain/PTControl Example/PTControl_In/CreateBus PTC ClutchIn ==
  In : Inport
  BusCreator : BusCreator  Inputs=6
  Demux : Demux  Outputs=6
  Out : Outport
  wires:
  In/1 -> Demux/1
  BusCreator/1 -> Out/1
  Demux/1 -> BusCreator/1  "PTC ClutchIn Pos"
  Demux/2 -> BusCreator/2  "PTC ClutchIn rotv_in"
  Demux/3 -> BusCreator/3  "PTC ClutchIn rotv_out"
  Demux/4 -> BusCreator/4  "PTC ClutchIn Trq_in"
  Demux/5 -> BusCreator/5  "PTC ClutchIn Trq_out"
  Demux/6 -> BusCreator/6  "PTC ClutchIn i_TrqIn2Out"

== system PTControl/CarMaker/IPG Vehicle/PowerTrain/PTControl Example/PTControl_In/CreateBus PTC Control Units ==
  In : Inport
  BusCreator : BusCreator
  Demux : Demux
  Out : Outport
  wires:
  In/1 -> Demux/1
  BusCreator/1 -> Out/1
  Demux/1 -> BusCreator/1  "PTC ECU_Status"
  Demux/2 -> BusCreator/2  "PTC MCU_Status"
  Demux/3 -> BusCreator/3  "PTC TCU_Status"
  Demux/4 -> BusCreator/4  "PTC BCU_Status"

== system PTControl/CarMaker/IPG Vehicle/PowerTrain/PTControl Example/PTControl_In/CreateBus PTC EngineIn ==
  In : Inport
  BusCreator : BusCreator  Inputs=7
  Demux : Demux  Outputs=7
  Out : Outport
  wires:
  Demux/7 -> BusCreator/7  "PTC EngineIn FuelFlow"
  In/1 -> Demux/1
  BusCreator/1 -> Out/1
  Demux/1 -> BusCreator/1  "PTC EngineIn Engine_on"
  Demux/2 -> BusCreator/2  "PTC EngineIn rotv"
  Demux/3 -> BusCreator/3  "PTC EngineIn Trq"
  Demux/4 -> BusCreator/4  "PTC EngineIn TrqDrag"
  Demux/5 -> BusCreator/5  "PTC EngineIn TrqFull"
  Demux/6 -> BusCreator/6  "PTC EngineIn TrqOpt"

== system PTControl/CarMaker/IPG Vehicle/PowerTrain/PTControl Example/PTControl_In/CreateBus PTC GearBoxIn ==
  In : Inport
  BusCreator : BusCreator  Inputs=13
  Demux : Demux  Outputs=13
  Out : Outport
  wires:
  In/1 -> Demux/1
  BusCreator/1 -> Out/1
  Demux/1 -> BusCreator/1  "PTC GearBoxIn GearNo"
  Demux/2 -> BusCreator/2  "PTC GearBoxIn Trq_in_off"
  Demux/3 -> BusCreator/3  "PTC GearBoxIn i"
  Demux/4 -> BusCreator/4  "PTC GearBoxIn rotv_in"
  Demux/5 -> BusCreator/5  "PTC GearBoxIn rotv_out"
  Demux/6 -> BusCreator/6  "PTC GearBoxIn Trq_in"
  Demux/7 -> BusCreator/7  "PTC GearBoxIn Trq_out"
  Demux/8 -> BusCreator/8  "PTC GearBoxIn Clutch Pos"
  Demux/9 -> BusCreator/9  "PTC GearBoxIn Clutch rotv_in"
  Demux/10 -> BusCreator/10  "PTC GearBoxIn Clutch rotv_out"
  Demux/11 -> BusCreator/11  "PTC GearBoxIn Clutch Trq_in"
  Demux/12 -> BusCreator/12  "PTC GearBoxIn Clutch Trq_out"
  Demux/13 -> BusCreator/13  "PTC GearBoxIn Clutch i_TrqIn2Out"

== system PTControl/CarMaker/IPG Vehicle/PowerTrain/PTControl Example/PTControl_In/CreateBus PTC GearBoxM_In0 ==
  In : Inport
  BusCreator : BusCreator  Inputs=13
  Demux : Demux  Outputs=13
  Out : Outport
  wires:
  In/1 -> Demux/1
  BusCreator/1 -> Out/1
  Demux/1 -> BusCreator/1  "PTC GearBoxM_In0 GearNo"
  Demux/2 -> BusCreator/2  "PTC GearBoxM_In0 Trq_in_off"
  Demux/3 -> BusCreator/3  "PTC GearBoxM_In0 i"
  Demux/4 -> BusCreator/4  "PTC GearBoxM_In0 rotv_in"
  Demux/5 -> BusCreator/5  "PTC GearBoxM_In0 rotv_out"
  Demux/6 -> BusCreator/6  "PTC GearBoxM_In0 Trq_in"
  Demux/7 -> BusCreator/7  "PTC GearBoxM_In0 Trq_out"
  Demux/8 -> BusCreator/8  "PTC GearBoxM_In0 Clutch Pos"
  Demux/9 -> BusCreator/9  "PTC GearBoxM_In0 Clutch rotv_in"
  Demux/10 -> BusCreator/10  "PTC GearBoxM_In0 Clutch rotv_out"
  Demux/11 -> BusCreator/11  "PTC GearBoxM_In0 Clutch Trq_in"
  Demux/12 -> BusCreator/12  "PTC GearBoxM_In0 Clutch Trq_out"
  Demux/13 -> BusCreator/13  "PTC GearBoxM_In0 Clutch i_TrqIn2Out"

== system PTControl/CarMaker/IPG Vehicle/PowerTrain/PTControl Example/PTControl_In/CreateBus PTC GearBoxM_In1 ==
  In : Inport
  BusCreator : BusCreator  Inputs=13
  Demux : Demux  Outputs=13
  Out : Outport
  wires:
  In/1 -> Demux/1
  BusCreator/1 -> Out/1
  Demux/1 -> BusCreator/1  "PTC GearBoxM_In1 GearNo"
  Demux/2 -> BusCreator/2  "PTC GearBoxM_In1 Trq_in_off"
  Demux/3 -> BusCreator/3  "PTC GearBoxM_In1 i"
  Demux/4 -> BusCreator/4  "PTC GearBoxM_In1 rotv_in"
  Demux/5 -> BusCreator/5  "PTC GearBoxM_In1 rotv_out"
  Demux/6 -> BusCreator/6  "PTC GearBoxM_In1 Trq_in"
  Demux/7 -> BusCreator/7  "PTC GearBoxM_In1 Trq_out"
  Demux/8 -> BusCreator/8  "PTC GearBoxM_In1 Clutch Pos"
  Demux/9 -> BusCreator/9  "PTC GearBoxM_In1 Clutch rotv_in"
  Demux/10 -> BusCreator/10  "PTC GearBoxM_In1 Clutch rotv_out"
  Demux/11 -> BusCreator/11  "PTC GearBoxM_In1 Clutch Trq_in"
  Demux/12 -> BusCreator/12  "PTC GearBoxM_In1 Clutch Trq_out"
  Demux/13 -> BusCreator/13  "PTC GearBoxM_In1 Clutch i_TrqIn2Out"

== system PTControl/CarMaker/IPG Vehicle/PowerTrain/PTControl Example/PTControl_In/CreateBus PTC GearBoxM_In2 ==
  In : Inport
  BusCreator : BusCreator  Inputs=13
  Demux : Demux  Outputs=13
  Out : Outport
  wires:
  In/1 -> Demux/1
  BusCreator/1 -> Out/1
  Demux/1 -> BusCreator/1  "PTC GearBoxM_In2 GearNo"
  Demux/2 -> BusCreator/2  "PTC GearBoxM_In2 Trq_in_off"
  Demux/3 -> BusCreator/3  "PTC GearBoxM_In2 i"
  Demux/4 -> BusCreator/4  "PTC GearBoxM_In2 rotv_in"
  Demux/5 -> BusCreator/5  "PTC GearBoxM_In2 rotv_out"
  Demux/6 -> BusCreator/6  "PTC GearBoxM_In2 Trq_in"
  Demux/7 -> BusCreator/7  "PTC GearBoxM_In2 Trq_out"
  Demux/8 -> BusCreator/8  "PTC GearBoxM_In2 Clutch Pos"
  Demux/9 -> BusCreator/9  "PTC GearBoxM_In2 Clutch rotv_in"
  Demux/10 -> BusCreator/10  "PTC GearBoxM_In2 Clutch rotv_out"
  Demux/11 -> BusCreator/11  "PTC GearBoxM_In2 Clutch Trq_in"
  Demux/12 -> BusCreator/12  "PTC GearBoxM_In2 Clutch Trq_out"
  Demux/13 -> BusCreator/13  "PTC GearBoxM_In2 Clutch i_TrqIn2Out"

== system PTControl/CarMaker/IPG Vehicle/PowerTrain/PTControl Example/PTControl_In/CreateBus PTC GearBoxM_In3 ==
  In : Inport
  BusCreator : BusCreator  Inputs=13
  Demux : Demux  Outputs=13
  Out : Outport
  wires:
  In/1 -> Demux/1
  BusCreator/1 -> Out/1
  Demux/1 -> BusCreator/1  "PTC GearBoxM_In3 GearNo"
  Demux/2 -> BusCreator/2  "PTC GearBoxM_In3 Trq_in_off"
  Demux/3 -> BusCreator/3  "PTC GearBoxM_In3 i"
  Demux/4 -> BusCreator/4  "PTC GearBoxM_In3 rotv_in"
  Demux/5 -> BusCreator/5  "PTC GearBoxM_In3 rotv_out"
  Demux/6 -> BusCreator/6  "PTC GearBoxM_In3 Trq_in"
  Demux/7 -> BusCreator/7  "PTC GearBoxM_In3 Trq_out"
  Demux/8 -> BusCreator/8  "PTC GearBoxM_In3 Clutch Pos"
  Demux/9 -> BusCreator/9  "PTC GearBoxM_In3 Clutch rotv_in"
  Demux/10 -> BusCreator/10  "PTC GearBoxM_In3 Clutch rotv_out"
  Demux/11 -> BusCreator/11  "PTC GearBoxM_In3 Clutch Trq_in"
  Demux/12 -> BusCreator/12  "PTC GearBoxM_In3 Clutch Trq_out"
  Demux/13 -> BusCreator/13  "PTC GearBoxM_In3 Clutch i_TrqIn2Out"

== system PTControl/CarMaker/IPG Vehicle/PowerTrain/PTControl Example/PTControl_In/CreateBus PTC ISGIn ==
  In : Inport
  BusCreator : BusCreator  Inputs=9
  Demux : Demux  Outputs=9
  Out : Outport
  wires:
  In/1 -> Demux/1
  BusCreator/1 -> Out/1
  Demux/1 -> BusCreator/1  "PTC ISGIn rotv"
  Demux/2 -> BusCreator/2  "PTC ISGIn Trq"
  Demux/3 -> BusCreator/3  "PTC ISGIn TrqMot_max"
  Demux/4 -> BusCreator/4  "PTC ISGIn TrqGen_max"
  Demux/5 -> BusCreator/5  "PTC ISGIn PwrElec"
  Demux/6 -> BusCreator/6  "PTC ISGIn i_M2W_FL"
  Demux/7 -> BusCreator/7  "PTC ISGIn i_M2W_FR"
  Demux/8 -> BusCreator/8  "PTC ISGIn i_M2W_RL"
  Demux/9 -> BusCreator/9  "PTC ISGIn i_M2W_RR"

== system PTControl/CarMaker/IPG Vehicle/PowerTrain/PTControl Example/PTControl_In/CreateBus PTC MotorIn0 ==
  In : Inport
  BusCreator : BusCreator  Inputs=9
  Demux : Demux  Outputs=9
  Out : Outport
  wires:
  In/1 -> Demux/1
  BusCreator/1 -> Out/1
  Demux/1 -> BusCreator/1  "PTC MotorIn0 rotv"
  Demux/2 -> BusCreator/2  "PTC MotorIn0 Trq"
  Demux/3 -> BusCreator/3  "PTC MotorIn0 TrqMot_max"
  Demux/4 -> BusCreator/4  "PTC MotorIn0 TrqGen_max"
  Demux/5 -> BusCreator/5  "PTC MotorIn0 PwrElec"
  Demux/6 -> BusCreator/6  "PTC MotorIn0 i_M2W_FL"
  Demux/7 -> BusCreator/7  "PTC MotorIn0 i_M2W_FR"
  Demux/8 -> BusCreator/8  "PTC MotorIn0 i_M2W_RL"
  Demux/9 -> BusCreator/9  "PTC MotorIn0 i_M2W_RR"

== system PTControl/CarMaker/IPG Vehicle/PowerTrain/PTControl Example/PTControl_In/CreateBus PTC MotorIn1 ==
  In : Inport
  BusCreator : BusCreator  Inputs=9
  Demux : Demux  Outputs=9
  Out : Outport
  wires:
  In/1 -> Demux/1
  BusCreator/1 -> Out/1
  Demux/1 -> BusCreator/1  "PTC MotorIn1 rotv"
  Demux/2 -> BusCreator/2  "PTC MotorIn1 Trq"
  Demux/3 -> BusCreator/3  "PTC MotorIn1 TrqMot_max"
  Demux/4 -> BusCreator/4  "PTC MotorIn1 TrqGen_max"
  Demux/5 -> BusCreator/5  "PTC MotorIn1 PwrElec"
  Demux/6 -> BusCreator/6  "PTC MotorIn1 i_M2W_FL"
  Demux/7 -> BusCreator/7  "PTC MotorIn1 i_M2W_FR"
  Demux/8 -> BusCreator/8  "PTC MotorIn1 i_M2W_RL"
  Demux/9 -> BusCreator/9  "PTC MotorIn1 i_M2W_RR"

== system PTControl/CarMaker/IPG Vehicle/PowerTrain/PTControl Example/PTControl_In/CreateBus PTC MotorIn2 ==
  In : Inport
  BusCreator : BusCreator  Inputs=9
  Demux : Demux  Outputs=9
  Out : Outport
  wires:
  In/1 -> Demux/1
  BusCreator/1 -> Out/1
  Demux/1 -> BusCreator/1  "PTC MotorIn2 rotv"
  Demux/2 -> BusCreator/2  "PTC MotorIn2 Trq"
  Demux/3 -> BusCreator/3  "PTC MotorIn2 TrqMot_max"
  Demux/4 -> BusCreator/4  "PTC MotorIn2 TrqGen_max"
  Demux/5 -> BusCreator/5  "PTC MotorIn2 PwrElec"
  Demux/6 -> BusCreator/6  "PTC MotorIn2 i_M2W_FL"
  Demux/7 -> BusCreator/7  "PTC MotorIn2 i_M2W_FR"
  Demux/8 -> BusCreator/8  "PTC MotorIn2 i_M2W_RL"
  Demux/9 -> BusCreator/9  "PTC MotorIn2 i_M2W_RR"

== system PTControl/CarMaker/IPG Vehicle/PowerTrain/PTControl Example/PTControl_In/CreateBus PTC MotorIn3 ==
  In : Inport
  BusCreator : BusCreator  Inputs=9
  Demux : Demux  Outputs=9
  Out : Outport
  wires:
  In/1 -> Demux/1
  BusCreator/1 -> Out/1
  Demux/1 -> BusCreator/1  "PTC MotorIn3 rotv"
  Demux/2 -> BusCreator/2  "PTC MotorIn3 Trq"
  Demux/3 -> BusCreator/3  "PTC MotorIn3 TrqMot_max"
  Demux/4 -> BusCreator/4  "PTC MotorIn3 TrqGen_max"
  Demux/5 -> BusCreator/5  "PTC MotorIn3 PwrElec"
  Demux/6 -> BusCreator/6  "PTC MotorIn3 i_M2W_FL"
  Demux/7 -> BusCreator/7  "PTC MotorIn3 i_M2W_FR"
  Demux/8 -> BusCreator/8  "PTC MotorIn3 i_M2W_RL"
  Demux/9 -> BusCreator/9  "PTC MotorIn3 i_M2W_RR"

== system PTControl/CarMaker/IPG Vehicle/PowerTrain/PTControl Example/PTControl_In/CreateBus PTC PwrSupplyIn ==
  In : Inport
  BusCreator : BusCreator  Inputs=12
  Demux : Demux  Outputs=12
  Out : Outport
  wires:
  In/1 -> Demux/1
  BusCreator/1 -> Out/1
  Demux/1 -> BusCreator/1  "PTC PwrSupplyIn Pwr_LV"
  Demux/2 -> BusCreator/2  "PTC PwrSupplyIn Pwr_HV1"
  Demux/3 -> BusCreator/3  "PTC PwrSupplyIn Pwr_HV2"
  Demux/4 -> BusCreator/4  "PTC PwrSupplyIn Voltage_LV"
  Demux/5 -> BusCreator/5  "PTC PwrSupplyIn Voltage_HV1"
  Demux/6 -> BusCreator/6  "PTC PwrSupplyIn Voltage_HV2"
  Demux/7 -> BusCreator/7  "PTC PwrSupplyIn Pwr_HV1toLV"
  Demux/8 -> BusCreator/8  "PTC PwrSupplyIn Pwr_HV1toHV2"
  Demux/9 -> BusCreator/9  "PTC PwrSupplyIn Pwr_HV1toLV_max"
  Demux/10 -> BusCreator/10  "PTC PwrSupplyIn Pwr_HV1toHV2_max"
  Demux/11 -> BusCreator/11  "PTC PwrSupplyIn Eta_HV1toLV"
  Demux/12 -> BusCreator/12  "PTC PwrSupplyIn Eta_HV1toHV2"

== system PTControl/CarMaker/IPG Vehicle/PowerTrain/PTControl Example/PTControl_In/CreateBus PTC WheelIn ==
  In : Inport
  BusCreator : BusCreator
  Demux : Demux
  Out : Outport
  wires:
  In/1 -> Demux/1
  BusCreator/1 -> Out/1
  Demux/1 -> BusCreator/1  "PTC WheelIn_FL Trq_BrakeReg_trg"
  Demux/2 -> BusCreator/2  "PTC WheelIn_FR Trq_BrakeReg_trg"
  Demux/3 -> BusCreator/3  "PTC WheelIn_RL Trq_BrakeReg_trg"
  Demux/4 -> BusCreator/4  "PTC WheelIn_RR Trq_BrakeReg_trg"

== system PTControl/CarMaker/IPG Vehicle/PowerTrain/PTControl Example/PTControl_In/CreateBus PTC_Cfg Battery ==
  In : Inport
  BusCreator : BusCreator  Inputs=8
  Demux : Demux  Outputs=8
  Out : Outport
  wires:
  In/1 -> Demux/1
  BusCreator/1 -> Out/1
  Demux/1 -> BusCreator/1  "PTC_Cfg BattLV SOC_min"
  Demux/2 -> BusCreator/2  "PTC_Cfg BattLV SOC_max"
  Demux/3 -> BusCreator/3  "PTC_Cfg BattLV Capacity"
  Demux/4 -> BusCreator/4  "PTC_Cfg BattLV Voltage"
  Demux/5 -> BusCreator/5  "PTC_Cfg BattHV SOC_min"
  Demux/6 -> BusCreator/6  "PTC_Cfg BattHV SOC_max"
  Demux/7 -> BusCreator/7  "PTC_Cfg BattHV Capacity"
  Demux/8 -> BusCreator/8  "PTC_Cfg BattHV Voltage"

== system PTControl/CarMaker/IPG Vehicle/PowerTrain/PTControl Example/PTControl_In/CreateBus PTC_Cfg Engine ==
  In : Inport
  BusCreator1 : BusCreator
  Demux1 : Demux
  Out : Outport
  wires:
  Demux1/1 -> BusCreator1/1  "PTC_Cfg Engine Fuel_l2kWh"
  Demux1/2 -> BusCreator1/2  "PTC_Cfg Engine rotv_max"
  Demux1/3 -> BusCreator1/3  "PTC_Cfg Engine rotv_idle"
  Demux1/4 -> BusCreator1/4  "PTC_Cfg Engine rotv_opt"
  In/1 -> Demux1/1
  BusCreator1/1 -> Out/1

== system PTControl/CarMaker/IPG Vehicle/PowerTrain/PTControl Example/PTControl_In/CreateBus PTC_Cfg GearBox ==
  In : Inport
  BusCreator : BusCreator  Inputs=38
  Demux : Demux  Outputs=38
  Out : Outport
  wires:
  In/1 -> Demux/1
  BusCreator/1 -> Out/1
  Demux/1 -> BusCreator/1  "PTC_Cfg GearBox GBKind"
  Demux/2 -> BusCreator/2  "PTC_Cfg GearBox ClKind"
  Demux/3 -> BusCreator/3  "PTC_Cfg GearBox nFGears"
  Demux/4 -> BusCreator/4  "PTC_Cfg GearBox iFGear0"
  Demux/5 -> BusCreator/5  "PTC_Cfg GearBox iFGear1"
  Demux/6 -> BusCreator/6  "PTC_Cfg GearBox iFGear2"
  Demux/7 -> BusCreator/7  "PTC_Cfg GearBox iFGear3"
  Demux/8 -> BusCreator/8  "PTC_Cfg GearBox iFGear4"
  Demux/9 -> BusCreator/9  "PTC_Cfg GearBox iFGear5"
  Demux/10 -> BusCreator/10  "PTC_Cfg GearBox iFGear6"
  Demux/11 -> BusCreator/11  "PTC_Cfg GearBox iFGear7"
  Demux/12 -> BusCreator/12  "PTC_Cfg GearBox iFGear8"
  Demux/13 -> BusCreator/13  "PTC_Cfg GearBox iFGear9"
  Demux/14 -> BusCreator/14  "PTC_Cfg GearBox iFGear10"
  Demux/15 -> BusCreator/15  "PTC_Cfg GearBox iFGear11"
  Demux/16 -> BusCreator/16  "PTC_Cfg GearBox iFGear12"
  Demux/17 -> BusCreator/17  "PTC_Cfg GearBox iFGear13"
  Demux/18 -> BusCreator/18  "PTC_Cfg GearBox iFGear14"
  Demux/19 -> BusCreator/19  "PTC_Cfg GearBox iFGear15"
  Demux/20 -> BusCreator/20  "PTC_Cfg GearBox iFGear16"
  Demux/21 -> BusCreator/21  "PTC_Cfg GearBox nBGears"
  Demux/22 -> BusCreator/22  "PTC_Cfg GearBox iBGear0"
  Demux/23 -> BusCreator/23  "PTC_Cfg GearBox iBGear1"
  Demux/24 -> BusCreator/24  "PTC_Cfg GearBox iBGear2"
  Demux/25 -> BusCreator/25  "PTC_Cfg GearBox iBGear3"
  Demux/26 -> BusCreator/26  "PTC_Cfg GearBox iBGear4"
  Demux/27 -> BusCreator/27  "PTC_Cfg GearBox iBGear5"
  Demux/28 -> BusCreator/28  "PTC_Cfg GearBox iBGear6"
  Demux/29 -> BusCreator/29  "PTC_Cfg GearBox iBGear7"
  Demux/30 -> BusCreator/30  "PTC_Cfg GearBox iBGear8"
  Demux/31 -> BusCreator/31  "PTC_Cfg GearBox iBGear9"
  Demux/32 -> BusCreator/32  "PTC_Cfg GearBox iBGear10"
  Demux/33 -> BusCreator/33  "PTC_Cfg GearBox iBGear11"
  Demux/34 -> BusCreator/34  "PTC_Cfg GearBox iBGear12"
  Demux/35 -> BusCreator/35  "PTC_Cfg GearBox iBGear13"
  Demux/36 -> BusCreator/36  "PTC_Cfg GearBox iBGear14"
  Demux/37 -> BusCreator/37  "PTC_Cfg GearBox iBGear15"
  Demux/38 -> BusCreator/38  "PTC_Cfg GearBox iBGear16"

== system PTControl/CarMaker/IPG Vehicle/PowerTrain/PTControl Example/PTControl_In/CreateBus PTC_Cfg GearBoxM0 ==
  In : Inport
  BusCreator : BusCreator  Inputs=38
  Demux : Demux  Outputs=38
  Out : Outport
  wires:
  In/1 -> Demux/1
  BusCreator/1 -> Out/1
  Demux/1 -> BusCreator/1  "PTC_Cfg GearBoxM0 GBKind"
  Demux/2 -> BusCreator/2  "PTC_Cfg GearBoxM0 ClKind"
  Demux/3 -> BusCreator/3  "PTC_Cfg GearBoxM0 nFGears"
  Demux/4 -> BusCreator/4  "PTC_Cfg GearBoxM0 iFGear0"
  Demux/5 -> BusCreator/5  "PTC_Cfg GearBoxM0 iFGear1"
  Demux/6 -> BusCreator/6  "PTC_Cfg GearBoxM0 iFGear2"
  Demux/7 -> BusCreator/7  "PTC_Cfg GearBoxM0 iFGear3"
  Demux/8 -> BusCreator/8  "PTC_Cfg GearBoxM0 iFGear4"
  Demux/9 -> BusCreator/9  "PTC_Cfg GearBoxM0 iFGear5"
  Demux/10 -> BusCreator/10  "PTC_Cfg GearBoxM0 iFGear6"
  Demux/11 -> BusCreator/11  "PTC_Cfg GearBoxM0 iFGear7"
  Demux/12 -> BusCreator/12  "PTC_Cfg GearBoxM0 iFGear8"
  Demux/13 -> BusCreator/13  "PTC_Cfg GearBoxM0 iFGear9"
  Demux/14 -> BusCreator/14  "PTC_Cfg GearBoxM0 iFGear10"
  Demux/15 -> BusCreator/15  "PTC_Cfg GearBoxM0 iFGear11"
  Demux/16 -> BusCreator/16  "PTC_Cfg GearBoxM0 iFGear12"
  Demux/17 -> BusCreator/17  "PTC_Cfg GearBoxM0 iFGear13"
  Demux/18 -> BusCreator/18  "PTC_Cfg GearBoxM0 iFGear14"
  Demux/19 -> BusCreator/19  "PTC_Cfg GearBoxM0 iFGear15"
  Demux/20 -> BusCreator/20  "PTC_Cfg GearBoxM0 iFGear16"
  Demux/21 -> BusCreator/21  "PTC_Cfg GearBoxM0 nBGears"
  Demux/22 -> BusCreator/22  "PTC_Cfg GearBoxM0 iBGear0"
  Demux/23 -> BusCreator/23  "PTC_Cfg GearBoxM0 iBGear1"
  Demux/24 -> BusCreator/24  "PTC_Cfg GearBoxM0 iBGear2"
  Demux/25 -> BusCreator/25  "PTC_Cfg GearBoxM0 iBGear3"
  Demux/26 -> BusCreator/26  "PTC_Cfg GearBoxM0 iBGear4"
  Demux/27 -> BusCreator/27  "PTC_Cfg GearBoxM0 iBGear5"
  Demux/28 -> BusCreator/28  "PTC_Cfg GearBoxM0 iBGear6"
  Demux/29 -> BusCreator/29  "PTC_Cfg GearBoxM0 iBGear7"
  Demux/30 -> BusCreator/30  "PTC_Cfg GearBoxM0 iBGear8"
  Demux/31 -> BusCreator/31  "PTC_Cfg GearBoxM0 iBGear9"
  Demux/32 -> BusCreator/32  "PTC_Cfg GearBoxM0 iBGear10"
  Demux/33 -> BusCreator/33  "PTC_Cfg GearBoxM0 iBGear11"
  Demux/34 -> BusCreator/34  "PTC_Cfg GearBoxM0 iBGear12"
  Demux/35 -> BusCreator/35  "PTC_Cfg GearBoxM0 iBGear13"
  Demux/36 -> BusCreator/36  "PTC_Cfg GearBoxM0 iBGear14"
  Demux/37 -> BusCreator/37  "PTC_Cfg GearBoxM0 iBGear15"
  Demux/38 -> BusCreator/38  "PTC_Cfg GearBoxM0 iBGear16"

== system PTControl/CarMaker/IPG Vehicle/PowerTrain/PTControl Example/PTControl_In/CreateBus PTC_Cfg GearBoxM1 ==
  In : Inport
  BusCreator : BusCreator  Inputs=38
  Demux : Demux  Outputs=38
  Out : Outport
  wires:
  In/1 -> Demux/1
  BusCreator/1 -> Out/1
  Demux/1 -> BusCreator/1  "PTC_Cfg GearBoxM1 GBKind"
  Demux/2 -> BusCreator/2  "PTC_Cfg GearBoxM1 ClKind"
  Demux/3 -> BusCreator/3  "PTC_Cfg GearBoxM1 nFGears"
  Demux/4 -> BusCreator/4  "PTC_Cfg GearBoxM1 iFGear0"
  Demux/5 -> BusCreator/5  "PTC_Cfg GearBoxM1 iFGear1"
  Demux/6 -> BusCreator/6  "PTC_Cfg GearBoxM1 iFGear2"
  Demux/7 -> BusCreator/7  "PTC_Cfg GearBoxM1 iFGear3"
  Demux/8 -> BusCreator/8  "PTC_Cfg GearBoxM1 iFGear4"
  Demux/9 -> BusCreator/9  "PTC_Cfg GearBoxM1 iFGear5"
  Demux/10 -> BusCreator/10  "PTC_Cfg GearBoxM1 iFGear6"
  Demux/11 -> BusCreator/11  "PTC_Cfg GearBoxM1 iFGear7"
  Demux/12 -> BusCreator/12  "PTC_Cfg GearBoxM1 iFGear8"
  Demux/13 -> BusCreator/13  "PTC_Cfg GearBoxM1 iFGear9"
  Demux/14 -> BusCreator/14  "PTC_Cfg GearBoxM1 iFGear10"
  Demux/15 -> BusCreator/15  "PTC_Cfg GearBoxM1 iFGear11"
  Demux/16 -> BusCreator/16  "PTC_Cfg GearBoxM1 iFGear12"
  Demux/17 -> BusCreator/17  "PTC_Cfg GearBoxM1 iFGear13"
  Demux/18 -> BusCreator/18  "PTC_Cfg GearBoxM1 iFGear14"
  Demux/19 -> BusCreator/19  "PTC_Cfg GearBoxM1 iFGear15"
  Demux/20 -> BusCreator/20  "PTC_Cfg GearBoxM1 iFGear16"
  Demux/21 -> BusCreator/21  "PTC_Cfg GearBoxM1 nBGears"
  Demux/22 -> BusCreator/22  "PTC_Cfg GearBoxM1 iBGear0"
  Demux/23 -> BusCreator/23  "PTC_Cfg GearBoxM1 iBGear1"
  Demux/24 -> BusCreator/24  "PTC_Cfg GearBoxM1 iBGear2"
  Demux/25 -> BusCreator/25  "PTC_Cfg GearBoxM1 iBGear3"
  Demux/26 -> BusCreator/26  "PTC_Cfg GearBoxM1 iBGear4"
  Demux/27 -> BusCreator/27  "PTC_Cfg GearBoxM1 iBGear5"
  Demux/28 -> BusCreator/28  "PTC_Cfg GearBoxM1 iBGear6"
  Demux/29 -> BusCreator/29  "PTC_Cfg GearBoxM1 iBGear7"
  Demux/30 -> BusCreator/30  "PTC_Cfg GearBoxM1 iBGear8"
  Demux/31 -> BusCreator/31  "PTC_Cfg GearBoxM1 iBGear9"
  Demux/32 -> BusCreator/32  "PTC_Cfg GearBoxM1 iBGear10"
  Demux/33 -> BusCreator/33  "PTC_Cfg GearBoxM1 iBGear11"
  Demux/34 -> BusCreator/34  "PTC_Cfg GearBoxM1 iBGear12"
  Demux/35 -> BusCreator/35  "PTC_Cfg GearBoxM1 iBGear13"
  Demux/36 -> BusCreator/36  "PTC_Cfg GearBoxM1 iBGear14"
  Demux/37 -> BusCreator/37  "PTC_Cfg GearBoxM1 iBGear15"
  Demux/38 -> BusCreator/38  "PTC_Cfg GearBoxM1 iBGear16"
